simulink model "Simulacaoponteh"  (R2016a)
settings: Solver=VariableStepAuto  StartTime=0.0  StopTime=10.0  RelTol=1e-3
libraries: fl_lib x5, elec_lib x4
settings Model: Creator=Wyctor  LastModifiedBy=Wyctor

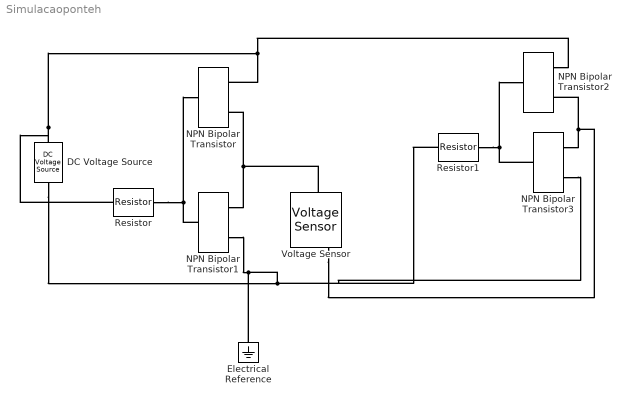
== system Simulacaoponteh ==
  DC Voltage Source : fl_lib/Electrical/Electrical Sources/DC Voltage Source  v0=1 V
  Electrical Reference : fl_lib/Electrical/Electrical Elements/Electrical Reference
  NPN Bipolar Transistor{,1..3} (4 alike) : elec_lib/Semiconductor Devices/NPN Bipolar Transistor  parameterization=1  prmDatasheet=1  prmEquCoeff=1  BF=100  IS=1e-14 A  ec=1  VAF=200 V  hfe=100  hoe=5e-5 1/Ohm  Ic_h=1 mA  Vce_h=5 V  V1=0.55 V  I1=0.5 mA  BR=1  Tmeas=25 degC  RC=0.01 Ohm  RE=1e-4 Ohm  RB=1 Ohm  C_BC=5 pF  C_BE=5 pF  TF=0 us  TR=0 us  hfe_T2=125  XTB=0  V1_T2=0.45 V  I1_T2=0.5 mA  Tmeas2=125 degC  EG=1.11 eV  XTI=3  TdeviceDatasheet=25 degC  TdeviceEquCoeff=25 degC  Rth=[ 0 10 ] K/W  thermal_mass_parameterization=1  thermal_mass=[ 0 1 ] J/K  thermal_time_constant=[ 0 10 ] s  thermal_mass_initial_temperatures=[ 25 25 ] degC
  Resistor : fl_lib/Electrical/Electrical Elements/Resistor  R=1 Ohm  i_specify=off  i_priority=None  i=0 A  v_specify=off  v_priority=None  v=0 V
  Resistor1 : fl_lib/Electrical/Electrical Elements/Resistor  R=1 Ohm  i_specify=off  i_priority=None  i=0 A  v_specify=off  v_priority=None  v=0 V
  Voltage Sensor : fl_lib/Electrical/Electrical Sensors/Voltage Sensor
  connections:
  NPN Bipolar Transistor1/RConn2 -- Resistor1/LConn1 -- NPN Bipolar Transistor3/RConn2 -- DC Voltage Source/RConn1 -- Electrical Reference/LConn1
  NPN Bipolar Transistor1/RConn1 -- Voltage Sensor/LConn1 -- NPN Bipolar Transistor/RConn2
  DC Voltage Source/LConn1 -- Resistor/LConn1 -- NPN Bipolar Transistor/RConn1 -- NPN Bipolar Transistor2/RConn1
  NPN Bipolar Transistor1/LConn1 -- NPN Bipolar Transistor/LConn1 -- Resistor/RConn1
  NPN Bipolar Transistor3/RConn1 -- Voltage Sensor/RConn2 -- NPN Bipolar Transistor2/RConn2
  NPN Bipolar Transistor3/LConn1 -- NPN Bipolar Transistor2/LConn1 -- Resistor1/RConn1
